simulink model "Ej5_model"  (R2018a)
settings: Solver=VariableStepAuto  StartTime=0.0  StopTime=10  RelTol=1e-3
values from neighbouring files (symbols this model uses):
  a = 200    [Ej1_params.m]    (also in Ej2_params.m; Ej3_params.m; Ej4_params.m; Ej5.m = results(i, 2))
  b = 10000    [Ej1_params.m]    (also in Ej2_params.m; Ej3_params.m; Ej4_params.m; Ej5.m = results(i, 3))
  K = results(i, 1)    [Ej5.m]
undefined symbols (not defined in the file or in its folder): N
settings Model: Creator=joses  LastModifiedBy=joses

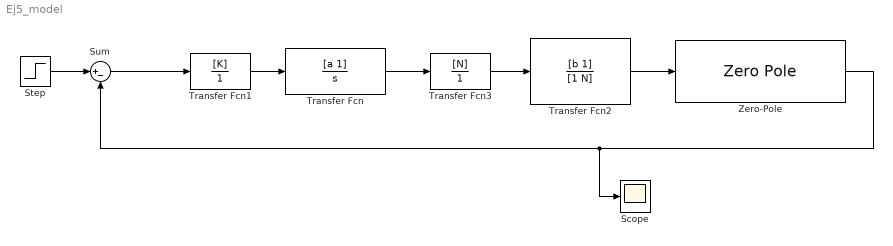
== system Ej5_model ==
  Scope : Scope
  Step : Step  SampleTime=0
  Sum : Sum  Inputs=|+-
  Transfer Fcn : TransferFcn  Numerator=[a 1]  Denominator=[1 0]
  Transfer Fcn1 : TransferFcn  Numerator=[K]  Denominator=[1]
  Transfer Fcn2 : TransferFcn  Numerator=[b 1]  Denominator=[1 N]
  Transfer Fcn3 : TransferFcn  Numerator=[N]  Denominator=[1]
  Zero-Pole : ZeroPole  Zeros=[-2]  Poles=[-10 -1]  Gain=2
  wires:
  Transfer Fcn1/1 -> Transfer Fcn/1
  Transfer Fcn/1 -> Transfer Fcn3/1
  Transfer Fcn2/1 -> Zero-Pole/1
  Sum/1 -> Transfer Fcn1/1
  Zero-Pole/1 -> Scope/1, Sum/2
  Step/1 -> Sum/1
  Transfer Fcn3/1 -> Transfer Fcn2/1
